simulink model "setpoint_model"  (R2023b)
settings: Solver=VariableStepAuto  StartTime=0.0  StopTime=10.0  RelTol=1e-3
values from neighbouring files (symbols this model uses):
  N_sp = size(setpoints,1)    [ddmr.m]    (also in simulaTrajetoriaSimulink.m)
  setpoints = readmatrix('../SETPOINTS/'+trajetoria+'.csv')    [testes2.m]
libraries: simulink x2
settings Model: Creator=Gabriel Sousa  LastModifiedBy=Gabriel Sousa

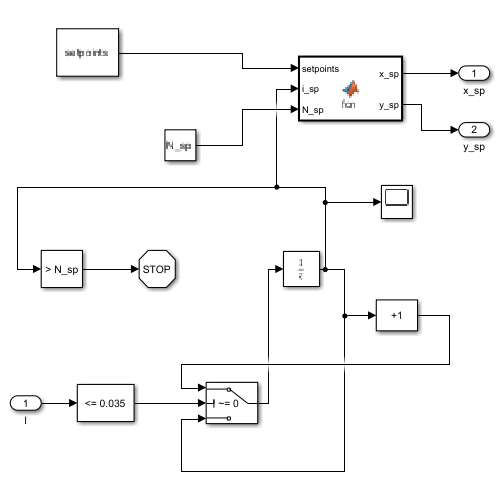
[thumbnail: Simulink's stored preview of the top-level diagram]
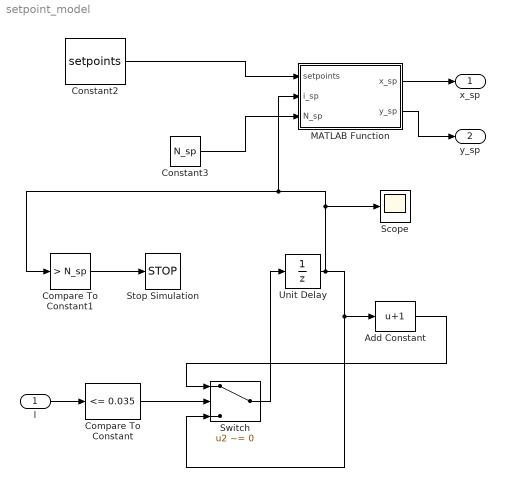
== system setpoint_model ==
  l : Inport
  Add Constant : Bias  Bias=1  SaturateOnIntegerOverflow=off
  Compare To Constant : simulink/Logic and Bit Operations/Compare To Constant  relop=<=  const=0.035  OutDataTypeStr=boolean
  Compare To Constant1 : simulink/Logic and Bit Operations/Compare To Constant  relop=>  const=N_sp  OutDataTypeStr=boolean
  Constant2 : Constant  Value=setpoints  VectorParams1D=off  OutDataTypeStr=single
  Constant3 : Constant  Value=N_sp
  MATLAB Function : MATLAB Function  TreatAsAtomicUnit=on
  Scope : Scope
  Stop Simulation : Stop
  Switch : Switch  Criteria=u2 ~= 0  SaturateOnIntegerOverflow=off  InputSameDT=off
  Unit Delay : UnitDelay  InitialCondition=2  SampleTime=-1  HasFrameUpgradeWarning=on
  x_sp : Outport
  y_sp : Outport  Port=2
  wires:
  Compare To Constant1/1 -> Stop Simulation/1
  MATLAB Function/1(x_sp) -> x_sp/1
  Compare To Constant/1 -> Switch/2
  Switch/1 -> Unit Delay/1
  MATLAB Function/2(y_sp) -> y_sp/1
  l/1 -> Compare To Constant/1
  Constant2/1 -> MATLAB Function/1(setpoints)
  Add Constant/1 -> Switch/1
  Unit Delay/1 -> Compare To Constant1/1, MATLAB Function/2(i_sp), Scope/1, Add Constant/1, Switch/3
  Constant3/1 -> MATLAB Function/3(N_sp)

== matlab function setpoint_model/MATLAB Function ==
  data: setpoints input; x_sp output; i_sp input; y_sp output; N_sp input
function [x_sp, y_sp] = fcn(setpoints,i_sp,N_sp)

if i_sp<1 || isempty(i_sp)
    i_sp = 1;
end
i_sp = int32(i_sp);
if i_sp<=N_sp
    x_sp = setpoints(i_sp,1);
    y_sp = setpoints(i_sp,2);
else
    x_sp = setpoints(end,1);
    y_sp = setpoints(end,2);

end
end
